simulink model "instancemerge"  (Simulink 6.6)
settings: Solver=FixedStepDiscrete  StartTime=0.0  StopTime=10.0  FixedStep=1  RelTol=1e-3
libraries: mergelibrary x3
settings Model: Creator=hnine  LastModifiedBy=hnine

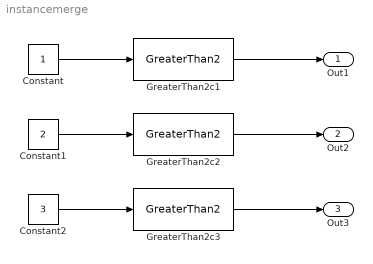
== system instancemerge ==
  Constant : Constant
  Constant1 : Constant  Value=2
  Constant2 : Constant  Value=3
  GreaterThan2c1 : mergelibrary/GreaterThan2  SystemSampleTime=-1
  GreaterThan2c2 : mergelibrary/GreaterThan2  SystemSampleTime=-1
  GreaterThan2c3 : mergelibrary/GreaterThan2  SystemSampleTime=-1
  Out1 : Outport
  Out2 : Outport  Port=2
  Out3 : Outport  Port=3
  wires:
  Constant/1 -> GreaterThan2c1/1
  Constant1/1 -> GreaterThan2c2/1
  Constant2/1 -> GreaterThan2c3/1
  GreaterThan2c1/1 -> Out1/1
  GreaterThan2c2/1 -> Out2/1
  GreaterThan2c3/1 -> Out3/1
